simulink library "coolant"  (R2022b)
settings: Solver=VariableStepAuto  StartTime=0.0  StopTime=10.0  RelTol=1e-3
undefined symbols (not defined in the file): raptor_xcp_function
libraries: Raptor_lib x6
settings Model: Creator=serga  LastModifiedBy=serga

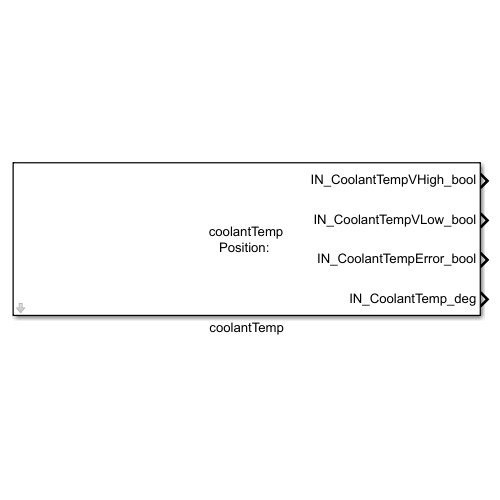
[thumbnail: Simulink's stored preview of the top-level diagram]
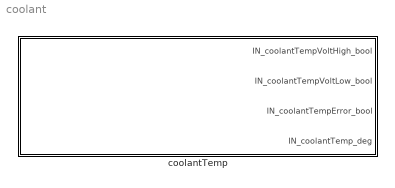
== system coolant ==
  coolantTemp : Subsystem  mask{pos=''}
      mask prompts: pos "Position"
      mask Display:
      | disp(['coolantTemp\n'...
      |     'Position: ' pos]);
      | port_label('output', 1, ['IN_' pos 'CoolantTempVHigh_bool']);
      | port_label('output', 2, ['IN_' pos 'CoolantTempVLow_bool']);
      | port_label('output', 3, ['IN_' pos 'CoolantTempError_bool']);
      | port_label('output', 4, ['IN_' pos 'CoolantTemp_deg']);

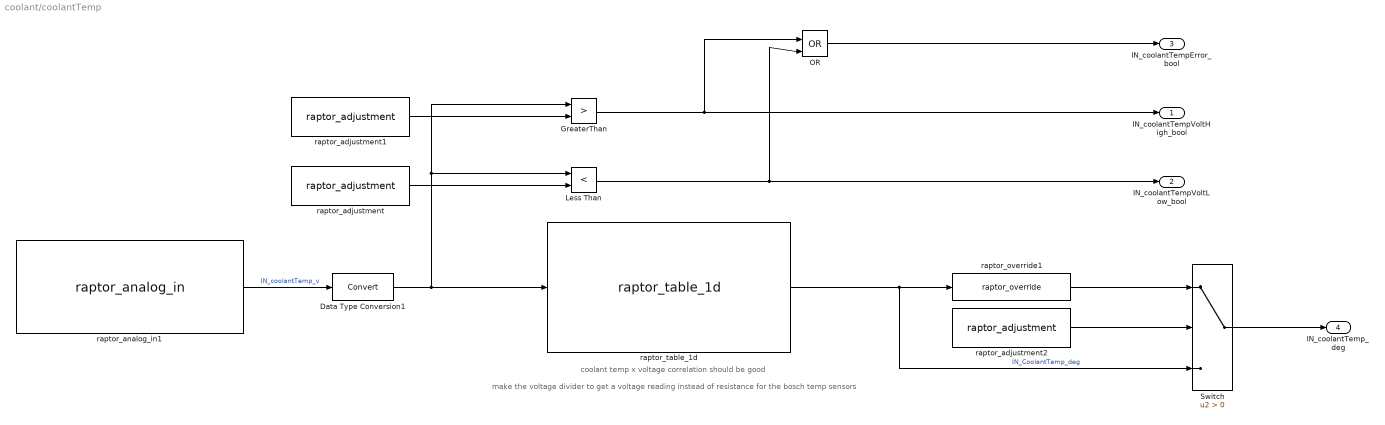
== system coolant/coolantTemp ==
  note: coolant temp x voltage correlation should be good
  note: make the voltage divider to get a voltage reading instead of resistance for the bosch temp sensors
  Data Type Conversion1 : DataTypeConversion  SaturateOnIntegerOverflow=off  RndMeth=Floor
  GreaterThan : RelationalOperator  Operator=>  OutDataTypeStr=boolean  RndMeth=Simplest  InputSameDT=off
  Less Than : RelationalOperator  Operator=<  OutDataTypeStr=boolean  RndMeth=Simplest  InputSameDT=off
  OR : Logic  Operator=OR  IconShape=distinctive  AllPortsSameDT=off  OutDataTypeStr=boolean
  Switch : Switch  Criteria=u2 > Threshold  SaturateOnIntegerOverflow=off  InputSameDT=off
  raptor_adjustment : Raptor_lib/Data Storage/raptor_adjustment  paramName=['IN_' pos 'CoolantTempLow_v']  nameSource=Parameter  initValue=0.5  dataType=single  storage=Calibration  calDispType=Number  calEnum={'False', 'True'}  calGain=1.0  calOffset=0.0  calMax=inf  calMin=-inf  calFormat='-1'  calUnit=''  calHelp=''  calAccess=1  calFunction=raptor_xcp_function(gcb)  calDispHeaders=off  calColHeaders={'Col1' 'Col2' 'Col3'}  calRowHeaders={'Row1' 'Row2' 'Row3'}
      settings: SourceProductName=Raptor
  raptor_adjustment1 : Raptor_lib/Data Storage/raptor_adjustment  paramName=['IN_' pos 'CoolantTempHigh_v']  nameSource=Parameter  initValue=4.5  dataType=single  storage=Calibration  calDispType=Number  calEnum={'False', 'True'}  calGain=1.0  calOffset=0.0  calMax=inf  calMin=-inf  calFormat='-1'  calUnit=''  calHelp=''  calAccess=1  calFunction=raptor_xcp_function(gcb)  calDispHeaders=off  calColHeaders={'Col1' 'Col2' 'Col3'}  calRowHeaders={'Row1' 'Row2' 'Row3'}
      settings: SourceProductName=Raptor
  raptor_adjustment2 : Raptor_lib/Data Storage/raptor_adjustment  paramName=['IN_' pos 'CoolantTemp_bool']  nameSource=Parameter  initValue=0.00  dataType=boolean  storage=Calibration  calDispType=Number  calEnum={'False', 'True'}  calGain=1.0  calOffset=0.0  calMax=inf  calMin=-inf  calFormat='-1'  calUnit=''  calHelp=''  calAccess=1  calFunction=raptor_xcp_function(gcb)  calDispHeaders=off  calColHeaders={'Col1' 'Col2' 'Col3'}  calRowHeaders={'Row1' 'Row2' 'Row3'}
      settings: SourceProductName=Raptor
  raptor_analog_in1 : Raptor_lib/Input & Output/raptor_analog_in  resourceValues=INPUT2|INPUT3|INPUT4|INPUT5|INPUT6|INPUT7|INPUT8|INPUT9|INPUT10|INPUT11|INPUT12|INPUT13|INPUT14|INPUT15|INPUT16|INPUT17|INPUT18|INPUT19|INPUT20|INPUT21|INPUT22|INPUT23|INPUT24|INPUT25|INPUT26|INPUT27|INPUT28|INPUT29|INPUT30|INPUT31|INPUT32|(None)  resource=INPUT2  pullUDValues=2.15k PU  pullUD=2.15k PU  rangeValues=0 - 5 V  range=0 - 5 V  filterrateValues=[]  filterrate='RAPTOR MASK DEFAULT'  resolutionValues=[]  resolution=[]
      settings: SourceProductName=Raptor
  raptor_override1 : Raptor_lib/Data Storage/raptor_override  paramName=['IN_' pos 'CoolantTemp_deg']  nameSource=Parameter  measurement=Output  calDispType=Number  calEnum={'False', 'True'}  calGain=1.0  calOffset=0.0  calMax=inf  calMin=-inf  calFormat='-1'  calUnit=''  calHelp=''  calAccess=1  calFunction="[raptor_xcp_function(gcb) '|'  'Override']"
      settings: SourceProductName=Raptor
  raptor_table_1d : Raptor_lib/Table Lookup/raptor_table_1d  dataName=['IN_' pos 'CoolantTempVToDeg']  initValue=[150 140 130 120 110 100 90 80 70 60 50 40 30 20 10 0 -10 -20 -30 -40]  dataType=single  storage=Calibration  initValueX=[0.2267 0.2793 0.3452 0.4303 0.5357 0.6741 0.8420 1.0604 1.3325 1.6592 2.0501 2.4737 2.9360 3.3784 3.7981 4.1545 4.4338 4.6399 4.7803 4.8710]  dataTypeXY=double  storageXY=Calibration  calVisible=on  showTable=on  calGain=1.0  calOffset=0.0  calMax=Inf  calMin=-Inf  calFormat='-1'  calUnit='Deg_C'  calHelp=''  showBreakpoint=on  dataNameX=[]  calGainX=1.0  calOffsetX=0.0  calMaxX=Inf  calMinX=-Inf  calFormatX='-1'  calUnitX='V'  calHelpX=''  calAccess=1  calFunction=raptor_xcp_function(gcb)  measureEnable=off  mName=['Data1D_Output']
      settings: SourceProductName=Raptor
  IN_coolantTempVoltHigh_bool : Outport
  IN_coolantTempVoltLow_bool : Outport  Port=2
  IN_coolantTempError_bool : Outport  Port=3
  IN_coolantTemp_deg : Outport  Port=4
  wires:
  raptor_override1/1 -> Switch/1
  OR/1 -> IN_coolantTempError_bool/1
  raptor_adjustment2/1 -> Switch/2
  raptor_analog_in1/1 -> Data Type Conversion1/1  "IN_coolantTemp_v"
  raptor_adjustment/1 -> Less Than/2
  raptor_table_1d/1 -> raptor_override1/1, Switch/3  "IN_CoolantTemp_deg"
  raptor_adjustment1/1 -> GreaterThan/2
  Switch/1 -> IN_coolantTemp_deg/1
  Less Than/1 -> IN_coolantTempVoltLow_bool/1, OR/2
  GreaterThan/1 -> OR/1, IN_coolantTempVoltHigh_bool/1
  Data Type Conversion1/1 -> GreaterThan/1, Less Than/1, raptor_table_1d/1
